simulink model "abort_logic_start"  (Simulink 8.0)
settings: Solver=ode3  StartTime=0.0  StopTime=3000  FixedStep=0.05  MaxStep=10  RelTol=1e-3
undefined symbols (not defined in the file): sigbuilder_block
libraries: simulink x1
settings Model: Creator=nicholas  LastModifiedBy=ZhouHaoyu
settings DataIOCC: SignalLoggingSaveFormat=ModelDataLogs
settings OptimizationCC: InitFltsAndDblsToZero=on
settings DebuggingCC: SaveWithParameterizedLinksMsg=none  SignalResolutionControl=TryResolveAllWithWarning  FcnCallInpInsideContextMsg=UseLocalSettings  StrictBusMsg=Warning
settings GRTTargetCC: TargetFcnLib=ansi_tfl_tmw.mat  CombineOutputUpdateFcns=off  GRTInterface=on

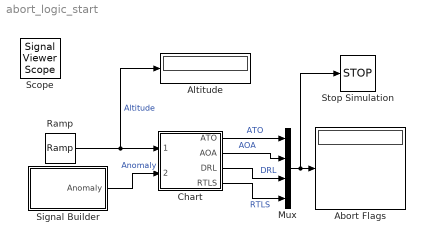
== system abort_logic_start ==
  Abort Flags : Display
  Altitude : Display
  Chart : Stateflow chart  TreatAsAtomicUnit=on
  Mux : Mux
  Ramp : simulink/Sources/Ramp  slope=20  start=0  X0=0
  Signal Builder : Subsystem  Tag=STV Subsys  LoadFcn=sigbuilder_block('load');  StartFcn=sigbuilder_block('start');  StopFcn=sigbuilder_block('stop');  ClipboardFcn=sigbuilder_block('clipboard');  mask(Sigbuilder block){}
      mask help: Sigbuilder GUI
      mask init:
      | if ~strcmp(get_param(bdroot(gcbh),'SimulationStatus'),'stopped') tuvar = sigbuilder_block('maskInit'); end
      settings: CopyFcn=sigbuilder_block('copy');  DeleteFcn=sigbuilder_block('delete');  ModelCloseFcn=sigbuilder_block('modelClose');  PreSaveFcn=sigbuilder_block('preSave');  PauseFcn=sigbuilder_block('pause')  ContinueFcn=sigbuilder_block('continue')  NameChangeFcn=sigbuilder_block('namechange');  OpenFcn=sigbuilder_block('open',[325.5 75 550.5 394.5 ]);  CloseFcn=sigbuilder_block('close');
      mask Display: plot(0,0,100,100,[10,10,40,40,10],[80,20,20,80,80],[40,10],[50,50], [40,27,10],[65,72,56],[40,25,25,10],[28,28,43,43]);
  Stop Simulation : Stop
  Scope : SignalViewerScope  IOType=viewer  RefreshTime=0.035000
  wires:
  Ramp/1 -> Chart/1(Altitude), Altitude/1  "Altitude"
  Chart/3(DRL) -> Mux/3  "DRL"
  Chart/4(RTLS) -> Mux/4  "RTLS"
  Mux/1 -> Abort Flags/1, Stop Simulation/1
  Chart/1(ATO) -> Mux/1  "ATO"
  Chart/2(AOA) -> Mux/2  "AOA"
  Signal Builder/1(Anomaly) -> Chart/2(Anormaly)  "Anomaly"

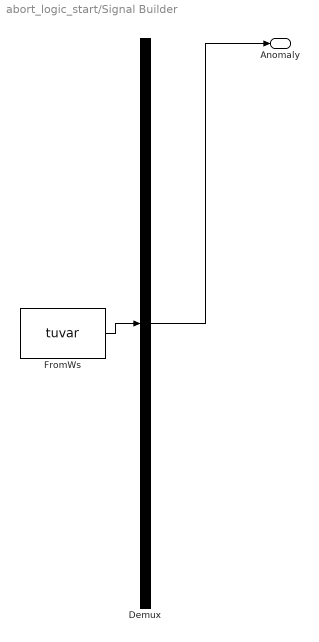
== system abort_logic_start/Signal Builder ==
  Demux : Demux  Tag=STV Demux  Outputs=1
  FromWs : FromWorkspace  Tag=STV FromWs  VariableName=tuvar  SampleTime=0  SigBuilderData=DataTag0  VnvData=DataTag1
      SigBuilderData=|
      | common.afterFinalStr = 'Extrapolate'
      | common.sampleTime = 0
      | dataSet(1).timeRange = [0 6000]
      | dataSet(1).name = 'RTLS'
      | dataSet(2).timeRange = [0 6000]
      | dataSet(2).name = 'DRL'
      | dataSet(3).timeRange = [0 6000]
      | dataSet(3).name = 'AOA'
      | dataSet(4).timeRange = [0 3000]
      | dataSet(4).name = 'ATO'
      | sbobj.Groups(1).Name = 'RTLS'
      | sbobj.Groups(1).Signals.Name = 'Anomaly'
      | sbobj.Groups(1).Signals.XData = [0 30 30 135 135 6000]
      | sbobj.Groups(1).Signals.YData = [0 0 1 1 0 0]
      | sbobj.Groups(1).TimeRange = [0 6000]
      | sbobj.Groups(2).Name = 'DRL'
      | sbobj.Groups(2).Signals.Name = 'Anomaly'
      | sbobj.Groups(2).Signals.XData = [0 250 250 340 340 6000]
      | sbobj.Groups(2).Signals.YData = [0 0 1 1 0 0]
      | sbobj.Groups(2).TimeRange = [0 6000]
      | sbobj.Groups(3).Name = 'AOA'
      | sbobj.Groups(3).Signals.Name = 'Anomaly'
      | sbobj.Groups(3).Signals.XData = [0 1005 1005 1100 1100 6000]
      | sbobj.Groups(3).Signals.YData = [0 0 1 1 0 0]
      | sbobj.Groups(3).TimeRange = [0 6000]
      | sbobj.Groups(4).Name = 'ATO'
      | sbobj.Groups(4).Signals.Name = 'Anomaly'
      | sbobj.Groups(4).Signals.XData = [0 2525 2525 2580 2580 3000]
      | sbobj.Groups(4).Signals.YData = [0 0 1 1 0 0]
      | sbobj.Groups(4).TimeRange = [0 3000]
  Anomaly : Outport  Tag=STV Outport
  wires:
  Demux/1 -> Anomaly/1
  FromWs/1 -> Demux/1

== stateflow chart Chart ==
  (default) -> (junction 9) : {ATO=0;AOA=0;DRL=0;}
  (junction 9) -> (junction 10) [order 1] : [Anormaly==1]
  (junction 10) -> (junction 11) [order 1] : [Altitude>=50000]
  (junction 9) -> (junction 16) [order 2]
  (junction 10) -> (junction 12) [order 2]
  (junction 11) -> (junction 20) : {ATO=1;}
  (junction 12) -> (junction 13) [order 1] : [Altitude>=10000]
  (junction 12) -> (junction 15) [order 2]
  (junction 13) -> (junction 19) : {AOA=1;}
  (junction 15) -> (junction 14) [order 1] : [Altitude>=1000]
  (junction 14) -> (junction 18) : {DRL=1;}
  (junction 15) -> (junction 17) [order 2] : {RTLS=1;}
  (junction 17) -> (junction 16)
  (junction 18) -> (junction 17)
  (junction 19) -> (junction 18)
  (junction 20) -> (junction 19)
  data: Altitude input double; Anormaly input double; ATO output double; AOA output double; DRL output double; RTLS output double
